simulink model "Kalman_Phase_NS_Double"  (R2019b)
settings: Solver=VariableStepAuto  StartTime=0.0  StopTime=phase_ns_model.sim_dur  FixedStep=model.Ts  RelTol=1e-6
undefined symbols (not defined in the file or in its folder): phase_ns_model
libraries: dspsrcs4 x11
settings Model: Creator=isidoraradenkovic  LastModifiedBy=isidoraradenkovic

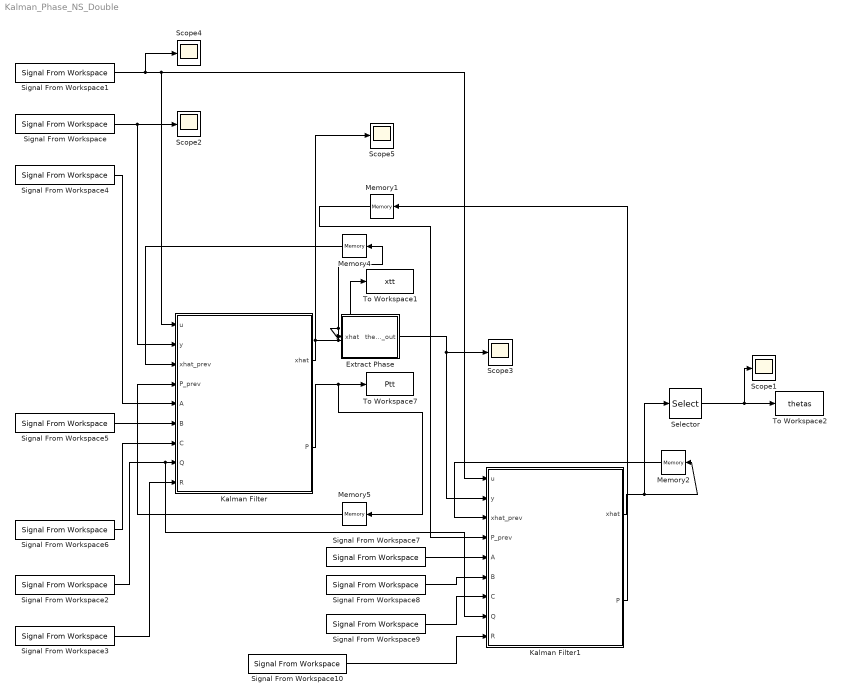
== system Kalman_Phase_NS_Double ==
  Extract Phase : MATLAB Function  TreatAsAtomicUnit=on  SystemSampleTime=phase_ns_model.Ts
  Kalman Filter : MATLAB Function  TreatAsAtomicUnit=on
  Kalman Filter1 : MATLAB Function  TreatAsAtomicUnit=on
  Memory1 : Memory  InitialCondition=phase_ns_model.P0  InheritSampleTime=on
  Memory2 : Memory  InitialCondition=phase_ns_model.x_0  InheritSampleTime=on
  Memory4 : Memory  InitialCondition=phase_ns_model.x_0  InheritSampleTime=on
  Memory5 : Memory  InitialCondition=phase_ns_model.P0  InheritSampleTime=on
  Scope{1..5} (5 alike) : Scope
  Selector : Selector  InputPortWidth=2  IndexOptions=Index vector (dialog)  Indices=[1]  OutputSizes=1
  Signal From Workspace : dspsrcs4/Signal From Workspace  X=input_data  Ts=phase_ns_model.Ts  nsamps=1  OutputAfterFinalValue=Cyclic repetition  ignoreOrWarnInputAndFrameLengths=off  OutputFrames=off
  Signal From Workspace1 : dspsrcs4/Signal From Workspace  X=tms_pulses  Ts=phase_ns_model.Ts  nsamps=1  OutputAfterFinalValue=Cyclic repetition  ignoreOrWarnInputAndFrameLengths=off  OutputFrames=off
  Signal From Workspace10 : dspsrcs4/Signal From Workspace  X=phase_double_model.R  Ts=phase_ns_model.Ts  nsamps=1  OutputAfterFinalValue=Cyclic repetition  ignoreOrWarnInputAndFrameLengths=off  OutputFrames=off
  Signal From Workspace2 : dspsrcs4/Signal From Workspace  X=phase_ns_model.Q  Ts=phase_ns_model.Ts/2  nsamps=2  OutputAfterFinalValue=Cyclic repetition  ignoreOrWarnInputAndFrameLengths=off  OutputFrames=off
  Signal From Workspace3 : dspsrcs4/Signal From Workspace  X=phase_ns_model.R  Ts=phase_ns_model.Ts  nsamps=1  OutputAfterFinalValue=Cyclic repetition  ignoreOrWarnInputAndFrameLengths=off  OutputFrames=off
  Signal From Workspace4 : dspsrcs4/Signal From Workspace  X=phase_ns_model.A  Ts=phase_ns_model.Ts/2  nsamps=2  OutputAfterFinalValue=Cyclic repetition  ignoreOrWarnInputAndFrameLengths=off  OutputFrames=off
  Signal From Workspace5 : dspsrcs4/Signal From Workspace  X=phase_ns_model.B  Ts=phase_ns_model.Ts/2  nsamps=2  OutputAfterFinalValue=Cyclic repetition  ignoreOrWarnInputAndFrameLengths=off  OutputFrames=off
  Signal From Workspace6 : dspsrcs4/Signal From Workspace  X=phase_ns_model.C  Ts=phase_ns_model.Ts  nsamps=1  OutputAfterFinalValue=Cyclic repetition  ignoreOrWarnInputAndFrameLengths=off  OutputFrames=off
  Signal From Workspace7 : dspsrcs4/Signal From Workspace  X=phase_double_model.A  Ts=phase_ns_model.Ts/2  nsamps=2  OutputAfterFinalValue=Cyclic repetition  ignoreOrWarnInputAndFrameLengths=off  OutputFrames=off
  Signal From Workspace8 : dspsrcs4/Signal From Workspace  X=phase_double_model.B  Ts=phase_ns_model.Ts/2  nsamps=2  OutputAfterFinalValue=Cyclic repetition  ignoreOrWarnInputAndFrameLengths=off  OutputFrames=off
  Signal From Workspace9 : dspsrcs4/Signal From Workspace  X=phase_double_model.C  Ts=phase_ns_model.Ts  nsamps=1  OutputAfterFinalValue=Cyclic repetition  ignoreOrWarnInputAndFrameLengths=off  OutputFrames=off
  To Workspace1 : ToWorkspace  VariableName=xtt  SampleTime=phase_ns_model.Ts
      settings: Save2DSignal=2-D array (concatenate along first dimension)
  To Workspace2 : ToWorkspace  VariableName=thetas  SampleTime=phase_ns_model.Ts
      settings: Save2DSignal=2-D array (concatenate along first dimension)
  To Workspace7 : ToWorkspace  VariableName=Ptt  SampleTime=phase_ns_model.Ts
      settings: Save2DSignal=2-D array (concatenate along first dimension)
  wires:
  Kalman Filter/2(P) -> To Workspace7/1, Memory5/1
  Signal From Workspace6/1 -> Kalman Filter/7(C)
  Signal From Workspace1/1 -> Kalman Filter1/1(u), Kalman Filter/1(u), Scope4/1
  Signal From Workspace3/1 -> Kalman Filter/9(R)
  Signal From Workspace2/1 -> Kalman Filter1/8(Q), Kalman Filter/8(Q)
  Signal From Workspace5/1 -> Kalman Filter/6(B)
  Kalman Filter/1(xhat) -> Scope5/1, Extract Phase/1(xhat), Memory4/1, To Workspace1/1
  Kalman Filter1/2(P) -> Memory1/1
  Signal From Workspace4/1 -> Kalman Filter/5(A)
  Extract Phase/1(thetas_out) -> Kalman Filter1/2(y), Scope3/1
  Memory4/1 -> Kalman Filter/3(xhat_prev)
  Kalman Filter1/1(xhat) -> Selector/1, Memory2/1
  Signal From Workspace/1 -> Scope2/1, Kalman Filter/2(y)
  Memory1/1 -> Kalman Filter1/4(P_prev)
  Memory5/1 -> Kalman Filter/4(P_prev)
  Memory2/1 -> Kalman Filter1/3(xhat_prev)
  Signal From Workspace7/1 -> Kalman Filter1/5(A)
  Signal From Workspace8/1 -> Kalman Filter1/6(B)
  Signal From Workspace9/1 -> Kalman Filter1/7(C)
  Signal From Workspace10/1 -> Kalman Filter1/9(R)
  Selector/1 -> To Workspace2/1, Scope1/1

== matlab function Kalman_Phase_NS_Double/Kalman Filter1 ==
  data: u input; xhat output; y input; xhat_prev input; P_prev input; A input; B input; C input; P output; Q input; R input
function [xhat, P] = clean_signal(u, y, xhat_prev, P_prev, A, B, C, Q, R)
x_time = A*xhat_prev;
P_time = A*P_prev*A'+ Q;

K = P_time*(C')*pinv(C*P_time*C' + R);
epsilon = y - C*x_time;

xhat = x_time + K*epsilon;
P = P_time - K*C*P_time;
end

== matlab function Kalman_Phase_NS_Double/Extract Phase ==
  settings: sampleTime=model.Ts
  data: xhat input; thetas_out output; phase_ns_model parameter
function thetas_out  = extract_phase(xhat, phase_ns_model)

thetas_out = mod(atan2(xhat(2), xhat(1))-2*pi*model.Ts*model.f-pi/2, 2*pi)-pi;

== matlab function Kalman_Phase_NS_Double/Kalman Filter ==
  data: u input; xhat output; y input; xhat_prev input; P_prev input; A input; B input; C input; P output; Q input; R input
function [xhat, P] = phase_ns_kalman(u, y, xhat_prev, P_prev, A, B, C, Q, R)
x_time = A*xhat_prev + B*u;
P_time = A*P_prev*A'+ Q;

K = P_time*(C')*pinv(C*P_time*C' + R);
epsilon = y - C*x_time;

xhat = x_time + K*epsilon;
P = P_time - K*C*P_time;
end
